simulink model "ex_16_model"  (R2014a)
settings: Solver=ode45  StartTime=0.0  StopTime=2  RelTol=1e-3
values from neighbouring files (symbols this model uses):
  G = 0    [ex_16_init.m]
  Kp = -1/(y/x)    (= 0.051)    [ex_16_init.m]    (also in ex_16_plot.m = 0.5*Kp0)
  x = -(1/J) * (a + (K^2/R))    (= -20.4)    [ex_16_init.m]
  y = (K/(J*R))    (= 400)    [ex_16_init.m]
  z = -(1/J)    (= -4000)    [ex_16_init.m]
settings Model: Creator=Nino  LastModifiedBy=Nino

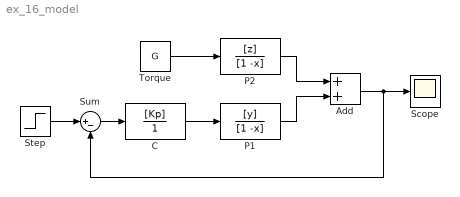
== system ex_16_model ==
  Add : Sum
  C : TransferFcn  Numerator=[Kp]  Denominator=[1]
  P1 : TransferFcn  Numerator=[y]  Denominator=[1 -x]
  P2 : TransferFcn  Numerator=[z]  Denominator=[1 -x]
  Scope : Scope
      settings: YMin=0.9989  YMax=0.9999  SaveName=Revolutions
  Step : Step  SampleTime=0
  Sum : Sum  Inputs=|+-
  Torque : Constant  Value=G
  wires:
  Torque/1 -> P2/1
  P2/1 -> Add/1
  P1/1 -> Add/2
  Add/1 -> Sum/2, Scope/1
  Step/1 -> Sum/1
  Sum/1 -> C/1
  C/1 -> P1/1
